simulink model "PIDController_1_r"  (Simulink 7.3)
settings: Solver=ode45  StartTime=0.0  StopTime=1  RelTol=1e-3
values from neighbouring files (symbols this model uses):
  Kd_gui = str2num(get(handles.edit6,'string'))    [Three_PID_Compare_noDistrup.m]    (also in Three_PID_Compare_withDistrup.m; changguiPID_noDistrup.m; changguiPID_withDistrup.m; mohuPID_noDistrup.m)
  Ki_gui = str2num(get(handles.edit5,'string'))    [Three_PID_Compare_noDistrup.m]    (also in Three_PID_Compare_withDistrup.m; changguiPID_noDistrup.m; changguiPID_withDistrup.m; mohuPID_noDistrup.m)
  Kp_gui = str2num(get(handles.edit4,'string'))    [Three_PID_Compare_noDistrup.m]    (also in Three_PID_Compare_withDistrup.m; changguiPID_noDistrup.m; changguiPID_withDistrup.m; mohuPID_noDistrup.m)
undefined symbols (not defined in the file or in its folder): sigbuilder_block
settings Model: Creator=Administrator  LastModifiedBy=Administrator

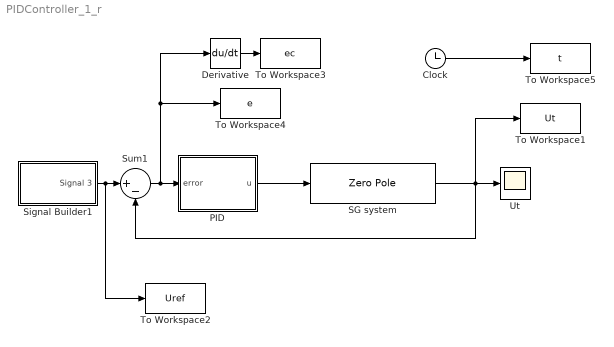
== system PIDController_1_r ==
  Clock : Clock
      settings: Decimation=10
  Derivative : Derivative
  PID : Subsystem  mask{Kp=Kp_gui, Ki=Ki_gui, Kd=Kd_gui}
      mask prompts: Kp "Proportional(Kp)"; Ki "Integral(Ki)"; Kd "Derivative(Kd)"
      mask help: Traditonal PID controller with three parameters:Proportional(Kp),Integral(Ki) and Derivative(Kd)
      mask Display: disp('PID Controller')
  SG system : ZeroPole  Zeros=[]  Poles=[-1/6 -20 -100]  Gain=20000
  Signal Builder1 : Subsystem  Tag=STV Subsys  LoadFcn=sigbuilder_block('load');  StartFcn=sigbuilder_block('start');  StopFcn=sigbuilder_block('stop');  ClipboardFcn=sigbuilder_block('clipboard');  mask(Sigbuilder block){}
      mask help: Sigbuilder GUI
      mask init:
      | if ~strcmp(get_param(bdroot(gcbh),'SimulationStatus'),'stopped') tuvar = sigbuilder_block('maskInit'); end
      settings: CopyFcn=sigbuilder_block('copy');  DeleteFcn=sigbuilder_block('delete');  ModelCloseFcn=sigbuilder_block('modelClose');  PreSaveFcn=sigbuilder_block('preSave');  NameChangeFcn=sigbuilder_block('namechange');  OpenFcn=sigbuilder_block('open',[3 45 954 496.5 ]);  CloseFcn=sigbuilder_block('close');
      mask Display: plot(0,0,100,100,[10,10,40,40,10],[80,20,20,80,80],[40,10],[50,50], [40,27,10],[65,72,56],[40,25,25,10],[28,28,43,43]);
  Sum1 : Sum  Inputs=|+-  OutDataType=sfix(16)  OutScaling=2^0
  To Workspace1 : ToWorkspace  VariableName=Ut  SampleTime=0.001  SaveFormat=Array
  To Workspace2 : ToWorkspace  VariableName=Uref  SampleTime=0.001  SaveFormat=Array
  To Workspace3 : ToWorkspace  VariableName=ec  SampleTime=0.001  SaveFormat=Array
  To Workspace4 : ToWorkspace  VariableName=e  SampleTime=0.001  SaveFormat=Array
  To Workspace5 : ToWorkspace  VariableName=t  SampleTime=0.001  SaveFormat=Array
  Ut : Scope
      settings: TimeRange=3  YMin=0  YMax=2
  wires:
  PID/1(u) -> SG system/1
  Signal Builder1/1(Signal 3) -> Sum1/1, To Workspace2/1
  Sum1/1 -> PID/1(error), To Workspace4/1, Derivative/1
  SG system/1 -> Ut/1, Sum1/2, To Workspace1/1
  Derivative/1 -> To Workspace3/1
  Clock/1 -> To Workspace5/1

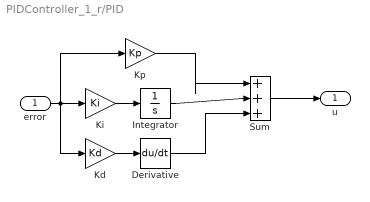
== system PIDController_1_r/PID ==
  error : Inport  OutDataType=fixdt(1, 16)  OutScaling=2^0
  Derivative : Derivative
  Integrator : Integrator
  Kd : Gain  Gain=Kd  ParameterDataType=fixdt(1, 16)  ParameterScaling=2^0  OutDataType=fixdt(1, 16)  OutScaling=2^0
  Ki : Gain  Gain=Ki  ParameterDataType=fixdt(1, 16)  ParameterScaling=2^0  OutDataType=fixdt(1, 16)  OutScaling=2^0
  Kp : Gain  Gain=Kp  ParameterDataType=fixdt(1, 16)  ParameterScaling=2^0  OutDataType=fixdt(1, 16)  OutScaling=2^0
  Sum : Sum  Inputs=|+++  OutDataType=fixdt(1, 16)  OutScaling=2^0
  u : Outport  OutDataType=fixdt(1, 16)  OutScaling=2^0
  wires:
  error/1 -> Kp/1, Ki/1, Kd/1
  Ki/1 -> Integrator/1
  Kd/1 -> Derivative/1
  Kp/1 -> Sum/1
  Integrator/1 -> Sum/2
  Derivative/1 -> Sum/3
  Sum/1 -> u/1

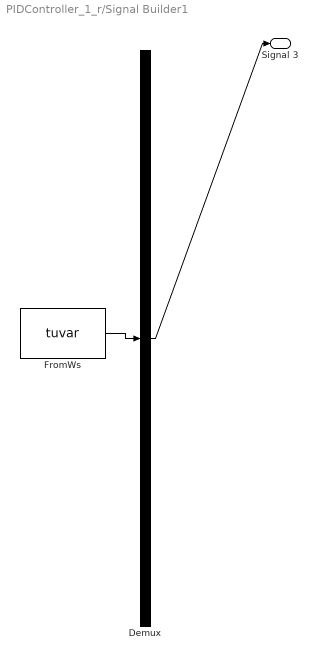
== system PIDController_1_r/Signal Builder1 ==
  Demux : Demux  Tag=STV Demux  Outputs=1
  FromWs : FromWorkspace  Tag=STV FromWs  VariableName=tuvar  SampleTime=0  SigBuilderData=DataTag0  VnvData=DataTag1
      SigBuilderData=|
      | common.afterFinalStr = 'Extrapolate'
      | common.sampleTime = 0
      | dataSet.timeRange = [0 1]
      | dataSet.name = 'Group 1'
      | sbobj.Groups.Signals.XData = [0 0.6 0.6 0.610526315789 0.621052631579 0.631578947368 0.642105263158 0.652631578947 0.663157894737 0.673684210526 0.684210526316 0.694736842105 0.705263157895 0.715789473684 0.726315789474 0.736842105263 0.747368421053 0.757894736842 0.768421052632 0.778947368421 0.789473684211 0.8 1]
      | sbobj.Groups.Signals.YData = [1 1 1 0.983540540972 0.96753005308 0.952405260696 0.938578728731 0.926427608933 0.916283352174 0.908422667334 0.903059973406 0.900341550699 0.900341550699 0.903059973406 0.908422667334 0.916283352174 0.926427608933 0.938578728731 0.952405260696 0.96753005308 0.983540540972 1 1]
  Signal 3 : Outport  Tag=STV Outport
  wires:
  FromWs/1 -> Demux/1
  Demux/1 -> Signal 3/1
